simulink model "project_RFT_DataGen2020a"  (R2020a)
settings: Solver=ode4  StartTime=0.0  StopTime=7  FixedStep=0.0001  MaxStep=1e-4  RelTol=1e-5
values from neighbouring files (symbols this model uses):
  Data = [0.0005 0.0005 0.0005 0.0005 0.0005 0.0005 0.0005 0.0005 0.0005 0.0005 0.0005 0.0005 ... (40000 elements, 10000x4)]    [Data.mat]    (also in DataGen2500.m = Data')
undefined symbols (not defined in the file or in its folder): i
settings Model: Creator=Mohamad Chehadeh  LastModifiedBy=mubar

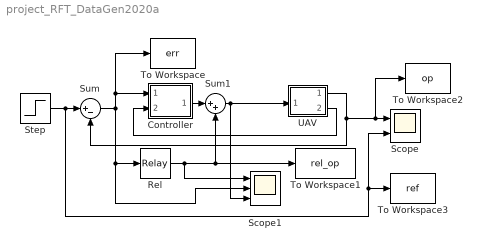
== system project_RFT_DataGen2020a ==
  Controller : Subsystem
  Rel : Relay  OffSwitchValue=-eps  OffOutputValue=-1
  Scope : Scope  NumInputPorts=2
  Scope1 : Scope  NumInputPorts=3
  Step : Step  SampleTime=0
  Sum : Sum  Inputs=|+-
  Sum1 : Sum  Inputs=|++
  To Workspace : ToWorkspace  VariableName=err  SaveFormat=Timeseries  SampleTime=-1
  To Workspace1 : ToWorkspace  VariableName=rel_op  SaveFormat=Timeseries  SampleTime=-1
  To Workspace2 : ToWorkspace  VariableName=op  SaveFormat=Timeseries  SampleTime=-1
  To Workspace3 : ToWorkspace  VariableName=ref  SaveFormat=Timeseries  SampleTime=-1
  UAV : Subsystem
  wires:
  Sum/1 -> Scope1/2, Rel/1, To Workspace/1, Controller/1(In1)
  UAV/1(Out1) -> Sum/2, To Workspace2/1, Scope/1
  UAV/2(Out2) -> Controller/2(In2)
  Controller/1(Out1) -> Sum1/1
  Rel/1 -> Scope1/1, To Workspace1/1, Sum1/2
  Step/1 -> Scope/2, To Workspace3/1, Sum/1
  Sum1/1 -> UAV/1(In1), Scope1/3

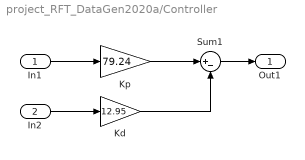
== system project_RFT_DataGen2020a/Controller ==
  In1 : Inport
  In2 : Inport  Port=2
  Kd : Gain  Gain=12.95
  Kp : Gain  Gain=79.24
  Sum1 : Sum  Inputs=|+-
  Out1 : Outport
  wires:
  In1/1 -> Kp/1
  Kp/1 -> Sum1/1
  In2/1 -> Kd/1
  Sum1/1 -> Out1/1
  Kd/1 -> Sum1/2

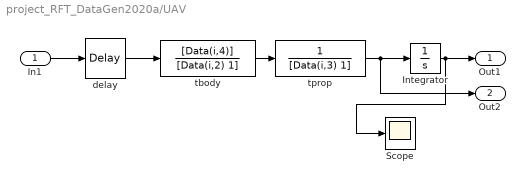
== system project_RFT_DataGen2020a/UAV ==
  In1 : Inport
  Integrator : Integrator
  Scope : Scope
  delay : TransportDelay  DelayTime=Data(i,1)
  tbody : TransferFcn  Numerator=[Data(i,4)]  Denominator=[Data(i,2) 1]
  tprop : TransferFcn  Denominator=[Data(i,3) 1]
  Out1 : Outport
  Out2 : Outport  Port=2
  wires:
  tbody/1 -> tprop/1
  In1/1 -> delay/1
  tprop/1 -> Out2/1, Integrator/1
  delay/1 -> tbody/1
  Integrator/1 -> Scope/1, Out1/1
